simulink model "nmpcSine"  (R2024b)
settings: Solver=FixedStepAuto  StartTime=0.0  StopTime=160  FixedStep=Ts  RelTol=1e-3
model workspace (MAT data in the model file):
  Logfile_Data_Object = ros2bag
  Logfile_Data_Object.FilePath = 'C:\Users\mpilo\Documents\Work\Research Project\Code\Catarob\ROS Implementation\Data\rosbag2_2024_09_20-12_24_11\rosbag2_2024_09_20-12_24_11_0.db3'
  Logfile_Data_Object.AvailableBags = "rosbag2_2024_09_20-12_24_11_0.db3"
  Logfile_Data_Object.StartTime = 1726827851.66
  Logfile_Data_Object.EndTime = 1726828062.45
  Logfile_Data_Object.AvailableTopics = table
  Logfile_Data_Object.AvailableTopics.data{1} = [653; 635; 211; 413; 21112]
  Logfile_Data_Object.AvailableTopics.data{2} = categorical
  Logfile_Data_Object.AvailableTopics.data{2}.categoryNames = {'catarob_interfaces/HullStatus'; 'sensor_msgs/Imu'; 'sensor_msgs/NavSatFix'; 'std_msgs/Float64'}
  Logfile_Data_Object.AvailableTopics.data{2}.codes = [1; 1; 3; 4; 2]
  Logfile_Data_Object.AvailableTopics.data{3}{1} = '
    | int32 status
    | single temp
    | int32 actual_pwm
    | int32 actual_pwm_rc
    | int32 pwm_source
    | single ibat
    | single imot
    | single vbat
    | single actual_imax
    | int32 tor_rc
    | int32 water_ingress
    | int32 pwr_relay'
  Logfile_Data_Object.AvailableTopics.data{3}{2} = '
    | int32 status
    | single temp
    | int32 actual_pwm
    | int32 actual_pwm_rc
    | int32 pwm_source
    | single ibat
    | single imot
    | single vbat
    | single actual_imax
    | int32 tor_rc
    | int32 water_ingress
    | int32 pwr_relay'
  Logfile_Data_Object.AvailableTopics.data{3}{3} = '%
    | % Specified using the WGS 84 reference ellipsoid
    | 
    | % header.stamp specifies the ROS Time for this measurement (the
    | %        corresponding satellite Time may be reported using the
    | %        sensor_msgs/TimeReference message).
    | %
    | % header.frame_id is the frame of reference reported by the satellite
    | %        receiver, usually the location of the antenna.  This is a
    | %        Euclidean frame relative to the vehicle, not a reference
    | %        ellipsoid.
    | std_msgs/Header header
    | 
    | % Satellite fix status information.
    | NavSatStatus status
    | 
    | % Latitude [degrees]. Positive is north of equator; negative is south.
    | double latitude
    | 
    | % Longitude [degrees]. Positive is east of prime meridian; negative is west.
    | double longitude
    | 
    | % Altitude [m]. Positive is above the WGS 84 ellipsoid
    | % (quiet NaN if no altitude is available).
    | double altitude
    | 
    | % Position covariance [m^2] defined relative to a tangential plane
    | % through the reported position. The components are East, North, and
    | % Up (ENU), in row-major order.
    | %
    | % Beware: this coordinate system exhibits singularities at the poles.
    | double[9] position_covariance
    | 
    | % If the covariance of the fix is known, fill it in completely. If the
    | % GPS receiver provides the variance of each measurement, put them
    | % along the diagonal. If only Dilution of Precision is available,
    | % estimate an approximate covariance from that.
    | 
    | uint8 COVARIANCE_TYPEUNKNOWN = 0
    | uint8 COVARIANCE_TYPEAPPROXIMATED = 1
    | uint8 COVARIANCE_TYPE_DIAGONALKNOWN = 2
    | uint8 COVARIANCE_TYPEKNOWN = 3
    | 
    | uint8 position_covariance_type'
  Logfile_Data_Object.AvailableTopics.data{3}{4} = '% It is deprecated as of Foxy
    | % It is recommended to create your own semantically meaningful message.
    | % However if you would like to continue using this please use the equivalent in example_msgs.
    | 
    | double data'
  Logfile_Data_Object.AvailableTopics.data{3}{5} = '%
    | % Accelerations should be in m/s^2 (not in g''s), and rotational velocity should be in rad/sec
    | %
    | % If the covariance of the measurement is known, it should be filled in (if all you know is the
    | % variance of each measurement, e.g. from the datasheet, just put those along the diagonal)
    | % A covariance matrix of all zeros will be interpreted as "covariance unknown", and to use the
    | % data a covariance will have to be assumed or gotten from some other source
    | %
    | % If you have no estimate for one of the data elements (e.g. your IMU doesn''t produce an
    | % orientation estimate), please set element 0 of the associated covariance matrix to -1
    | % If you are interpreting this message, please check for a value of -1 in the first element of each
    | % covariance matrix, and disregard the associated estimate.
    | 
    | std_msgs/Header header
    | 
    | geometry_msgs/Quaternion orientation
    | double[9] orientation_covariance         % Row major about x, y, z axes
    | 
    | geometry_msgs/Vector3 angular_velocity
    | double[9] angular_velocity_covariance    % Row major about x, y, z axes
    | 
    | geometry_msgs/Vector3 linear_acceleration
    | double[9] linear_acceleration_covariance % Row major x, y z'
  Logfile_Data_Object.AvailableTopics.ndims = 2
  Logfile_Data_Object.AvailableTopics.nrows = 5
  Logfile_Data_Object.AvailableTopics.rownames = {'/platform/hull/PORT_status'; '/platform/hull/STBD_status'; '/sensor/emlid_gps_fix'; '/sensors/mag_heading'; '/sensors/ouster/imu'}
  Logfile_Data_Object.AvailableTopics.nvars = 3
  Logfile_Data_Object.AvailableTopics.varnames = {'NumMessages', 'MessageType', 'MessageDefinition'}
  Logfile_Data_Object.AvailableTopics.props.useVariableNamesOriginal = 0
  Logfile_Data_Object.AvailableTopics.props.useDimensionNamesOriginal = 0
  Logfile_Data_Object.AvailableTopics.props.CustomProps = struct()
  Logfile_Data_Object.AvailableTopics.props.VariableCustomProps = struct()
  Logfile_Data_Object.AvailableTopics.props.versionSavedFrom = 4
  Logfile_Data_Object.AvailableTopics.props.minCompatibleVersion = 1
  Logfile_Data_Object.AvailableTopics.props.incompatibilityMsg = ''
  Logfile_Data_Object.AvailableTopics.props.VersionSavedFrom = 4
  Logfile_Data_Object.AvailableTopics.props.Description = ''
  Logfile_Data_Object.AvailableTopics.props.VariableNamesOriginal = {}
  Logfile_Data_Object.AvailableTopics.props.DimensionNames = {'Row', 'Variables'}
  Logfile_Data_Object.AvailableTopics.props.DimensionNamesOriginal = {}
  Logfile_Data_Object.AvailableTopics.props.UserData = []
  Logfile_Data_Object.AvailableTopics.props.VariableDescriptions = {}
  Logfile_Data_Object.AvailableTopics.props.VariableUnits = {}
  Logfile_Data_Object.AvailableTopics.props.VariableContinuity = {}
  Logfile_Data_Object.MessageList = table
  Logfile_Data_Object.MessageList.data{1} = [1726827851.66 1726827851.66 1726827851.67 1726827851.67 1726827851.68 1726827851.69 1726827851.69 1726827851.69 1726827851.7 1726827851.7 1726827851.72 1726827851.72 ... (23024 elements, 23024x1)]
  Logfile_Data_Object.MessageList.data{2} = categorical
  Logfile_Data_Object.MessageList.data{2}.categoryNames = {'/platform/hull/PORT_status'; '/platform/hull/STBD_status'; '/sensor/emlid_gps_fix'; '/sensors/mag_heading'; '/sensors/ouster/imu'}
  Logfile_Data_Object.MessageList.data{2}.codes = [5 5 5 5 5 5 5 5 5 5 5 5 ... (23024 elements, 23024x1)]
  Logfile_Data_Object.MessageList.data{3} = categorical
  Logfile_Data_Object.MessageList.data{3}.categoryNames = {'catarob_interfaces/HullStatus'; 'sensor_msgs/NavSatFix'; 'std_msgs/Float64'; 'sensor_msgs/Imu'}
  Logfile_Data_Object.MessageList.data{3}.codes = [4 4 4 4 4 4 4 4 4 4 4 4 ... (23024 elements, 23024x1)]
  Logfile_Data_Object.MessageList.ndims = 2
  Logfile_Data_Object.MessageList.nrows = 23024
  Logfile_Data_Object.MessageList.nvars = 3
  Logfile_Data_Object.MessageList.varnames = {'Time', 'Topic', 'MessageType'}
  Logfile_Data_Object.MessageList.props.useVariableNamesOriginal = 0
  Logfile_Data_Object.MessageList.props.useDimensionNamesOriginal = 0
  Logfile_Data_Object.MessageList.props.CustomProps = struct()
  Logfile_Data_Object.MessageList.props.VariableCustomProps = struct()
  Logfile_Data_Object.MessageList.props.versionSavedFrom = 4
  Logfile_Data_Object.MessageList.props.minCompatibleVersion = 1
  Logfile_Data_Object.MessageList.props.incompatibilityMsg = ''
  Logfile_Data_Object.MessageList.props.VersionSavedFrom = 4
  Logfile_Data_Object.MessageList.props.Description = ''
  Logfile_Data_Object.MessageList.props.VariableNamesOriginal = {}
  Logfile_Data_Object.MessageList.props.DimensionNames = {'Row', 'Variables'}
  Logfile_Data_Object.MessageList.props.DimensionNamesOriginal = {}
  Logfile_Data_Object.MessageList.props.UserData = []
  Logfile_Data_Object.MessageList.props.VariableDescriptions = {}
  Logfile_Data_Object.MessageList.props.VariableUnits = {}
  Logfile_Data_Object.MessageList.props.VariableContinuity = {}
  Logfile_Data_Object.TopicTypeMap = containers.Map
  Logfile_Data_Object.TopicTypeMap.serialization.keys = {'/platform/hull/PORT_status', '/platform/hull/STBD_status', '/sensor/emlid_gps_fix', '/sensors/mag_heading', '/sensors/ouster/imu'}
  Logfile_Data_Object.TopicTypeMap.serialization.values = {'catarob_interfaces/HullStatus', 'catarob_interfaces/HullStatus', 'sensor_msgs/NavSatFix', 'std_msgs/Float64', 'sensor_msgs/Imu'}
  Logfile_Data_Object.TopicTypeMap.serialization.uniformity = 1
  Logfile_Data_Object.TopicTypeMap.serialization.keyType = 'char'
  Logfile_Data_Object.TopicTypeMap.serialization.valueType = 'char'
  Logfile_Data_Object.TopicDefinitionMap = containers.Map
  Logfile_Data_Object.TopicDefinitionMap.serialization.keys = {'/platform/hull/PORT_status', '/platform/hull/STBD_status', '/sensor/emlid_gps_fix', '/sensors/mag_heading', '/sensors/ouster/imu'}
  Logfile_Data_Object.TopicDefinitionMap.serialization.values{1} = '
    | int32 status
    | single temp
    | int32 actual_pwm
    | int32 actual_pwm_rc
    | int32 pwm_source
    | single ibat
    | single imot
    | single vbat
    | single actual_imax
    | int32 tor_rc
    | int32 water_ingress
    | int32 pwr_relay'
  Logfile_Data_Object.TopicDefinitionMap.serialization.values{2} = '
    | int32 status
    | single temp
    | int32 actual_pwm
    | int32 actual_pwm_rc
    | int32 pwm_source
    | single ibat
    | single imot
    | single vbat
    | single actual_imax
    | int32 tor_rc
    | int32 water_ingress
    | int32 pwr_relay'
  Logfile_Data_Object.TopicDefinitionMap.serialization.values{3} = '%
    | % Specified using the WGS 84 reference ellipsoid
    | 
    | % header.stamp specifies the ROS Time for this measurement (the
    | %        corresponding satellite Time may be reported using the
    | %        sensor_msgs/TimeReference message).
    | %
    | % header.frame_id is the frame of reference reported by the satellite
    | %        receiver, usually the location of the antenna.  This is a
    | %        Euclidean frame relative to the vehicle, not a reference
    | %        ellipsoid.
    | std_msgs/Header header
    | 
    | % Satellite fix status information.
    | NavSatStatus status
    | 
    | % Latitude [degrees]. Positive is north of equator; negative is south.
    | double latitude
    | 
    | % Longitude [degrees]. Positive is east of prime meridian; negative is west.
    | double longitude
    | 
    | % Altitude [m]. Positive is above the WGS 84 ellipsoid
    | % (quiet NaN if no altitude is available).
    | double altitude
    | 
    | % Position covariance [m^2] defined relative to a tangential plane
    | % through the reported position. The components are East, North, and
    | % Up (ENU), in row-major order.
    | %
    | % Beware: this coordinate system exhibits singularities at the poles.
    | double[9] position_covariance
    | 
    | % If the covariance of the fix is known, fill it in completely. If the
    | % GPS receiver provides the variance of each measurement, put them
    | % along the diagonal. If only Dilution of Precision is available,
    | % estimate an approximate covariance from that.
    | 
    | uint8 COVARIANCE_TYPEUNKNOWN = 0
    | uint8 COVARIANCE_TYPEAPPROXIMATED = 1
    | uint8 COVARIANCE_TYPE_DIAGONALKNOWN = 2
    | uint8 COVARIANCE_TYPEKNOWN = 3
    | 
    | uint8 position_covariance_type'
  Logfile_Data_Object.TopicDefinitionMap.serialization.values{4} = '% It is deprecated as of Foxy
    | % It is recommended to create your own semantically meaningful message.
    | % However if you would like to continue using this please use the equivalent in example_msgs.
    | 
    | double data'
  Logfile_Data_Object.TopicDefinitionMap.serialization.values{5} = '%
    | % Accelerations should be in m/s^2 (not in g''s), and rotational velocity should be in rad/sec
    | %
    | % If the covariance of the measurement is known, it should be filled in (if all you know is the
    | % variance of each measurement, e.g. from the datasheet, just put those along the diagonal)
    | % A covariance matrix of all zeros will be interpreted as "covariance unknown", and to use the
    | % data a covariance will have to be assumed or gotten from some other source
    | %
    | % If you have no estimate for one of the data elements (e.g. your IMU doesn''t produce an
    | % orientation estimate), please set element 0 of the associated covariance matrix to -1
    | % If you are interpreting this message, please check for a value of -1 in the first element of each
    | % covariance matrix, and disregard the associated estimate.
    | 
    | std_msgs/Header header
    | 
    | geometry_msgs/Quaternion orientation
    | double[9] orientation_covariance         % Row major about x, y, z axes
    | 
    | geometry_msgs/Vector3 angular_velocity
    | double[9] angular_velocity_covariance    % Row major about x, y, z axes
    | 
    | geometry_msgs/Vector3 linear_acceleration
    | double[9] linear_acceleration_covariance % Row major x, y z'
  Logfile_Data_Object.TopicDefinitionMap.serialization.uniformity = 1
  Logfile_Data_Object.TopicDefinitionMap.serialization.keyType = 'char'
  Logfile_Data_Object.TopicDefinitionMap.serialization.valueType = 'char'
  Logfile_Data_Object.RawMessageBuffer = containers.Map
  Logfile_Data_Object.RawMessageBuffer.serialization.keys = {}
  Logfile_Data_Object.RawMessageBuffer.serialization.values = {}
  Logfile_Data_Object.RawMessageBuffer.serialization.uniformity = 0
  Logfile_Data_Object.RawMessageBuffer.serialization.keyType = 'char'
  Logfile_Data_Object.RawMessageBuffer.serialization.valueType = 'any'
  Logfile_Data_Object.ImgMessageBuffer = containers.Map
  Logfile_Data_Object.ImgMessageBuffer.serialization.keys = {}
  Logfile_Data_Object.ImgMessageBuffer.serialization.values = {}
  Logfile_Data_Object.ImgMessageBuffer.serialization.uniformity = 0
  Logfile_Data_Object.ImgMessageBuffer.serialization.keyType = 'char'
  Logfile_Data_Object.ImgMessageBuffer.serialization.valueType = 'any'
  Logfile_Data_Object.PointCloudBuffer = containers.Map
  Logfile_Data_Object.PointCloudBuffer.serialization.keys = {}
  Logfile_Data_Object.PointCloudBuffer.serialization.values = {}
  Logfile_Data_Object.PointCloudBuffer.serialization.uniformity = 0
  Logfile_Data_Object.PointCloudBuffer.serialization.keyType = 'char'
  Logfile_Data_Object.PointCloudBuffer.serialization.valueType = 'any'
  Logfile_Data_Object.LaserScanBuffer = containers.Map
  Logfile_Data_Object.LaserScanBuffer.serialization.keys = {}
  Logfile_Data_Object.LaserScanBuffer.serialization.values = {}
  Logfile_Data_Object.LaserScanBuffer.serialization.uniformity = 0
  Logfile_Data_Object.LaserScanBuffer.serialization.keyType = 'char'
  Logfile_Data_Object.LaserScanBuffer.serialization.valueType = 'any'
  Logfile_Path = 'C:\Users\mpilo\Documents\Work\Research Project\Code\Catarob\ROS Implementation\Data\rosbag2_2024_09_20-12_24_11\rosbag2_2024_09_20-12_24_11_0.db3'
  Logfile_Playback_Duration = nan
  Logfile_Playback_Offset = nan
values from neighbouring files (symbols this model uses):
  x = X(2:p+1,1)    [costFcn.m]    (also in costFcnJacobian.m = X(2:p+1, 1); stateTransitionFcnJacobianAD.m = x(:))
  y = [x(1);x(2);x(3);x(6)]    [SystemDynamics.m]    (also in costFcn.m = X(2:p+1,2); costFcnJacobian.m = X(2:p+1, 2); gpsMeasurementFcn.m = x([1 2]); imuMeasurementFcn.m = x(6))
undefined symbols (not defined in the file or in its folder): angular, covariance, linear, psi, r, regMdl, Ts, Ts_gps, Ts_mag, v, x_ref2, y_ref2
libraries: ros2lib x12, sharedTrackingLibrary x1, mpclib x1
settings Model: Creator=mpilo  LastModifiedBy=mpilo
settings OptimizationCC: DefaultParameterBehavior=Inlined  EnhancedBackFolding=on  PassReuseOutputArgsAs=Individual arguments  ZeroExternalMemoryAtStartup=off  ZeroInternalMemoryAtStartup=off  MaxStackSize=64  OptimizeBlockOrder=speed  DifferentSizesBufferReuse=on  OptimizationCustomize=off  EfficientTunableParamExpr=on
settings DebuggingCC: ParameterTunabilityLossMsg=error
settings HardwareCC: ProdBitPerLong=64  ProdHWDeviceType=Intel->x86-64 (Linux 64)
settings SFSimCC: MATLABDynamicMemAlloc=off
settings RTWCC: Description=Embedded Coder  SystemTargetFile=ert.tlc  HardwareBoard=Robot Operating System 2 (ROS 2)  TLCOptions="-aInlineSetEventsForThisBaseRateFcn=TLC_FALSE -aSuppressMultiTaskScheduler=TLC_FALSE  -aRateBasedStepFcn=0"  TemplateMakefile=ert_default_tmf  Toolchain=Colcon Tools  TargetLang=C++
settings CodeAppCC: ForceParamTrailComments=on  IgnoreCustomStorageClasses=off  OperatorAnnotations=on  SimulinkDataObjDesc=on  SFDataObjDesc=on  InsertBlockDesc=on
settings ERTTargetCC: CodeInterfacePackaging=C++ class  SupportComplex=off  SupportVariableSizeSignals=on  RootIOFormat=Structure reference

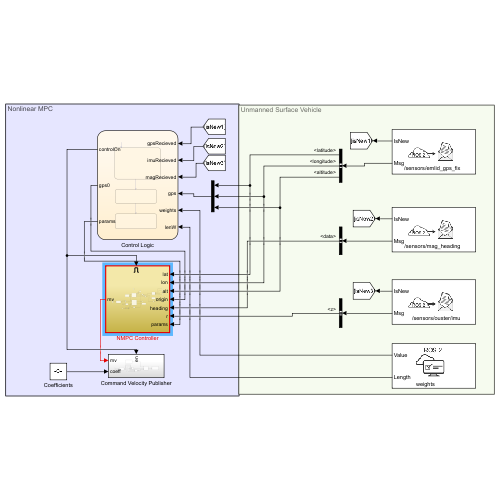
[thumbnail: Simulink's stored preview of the top-level diagram]
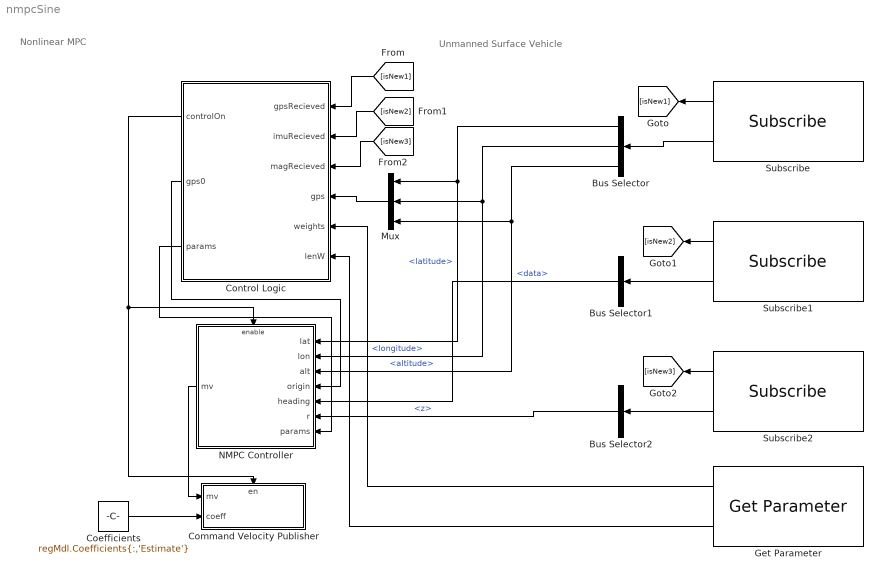
== system nmpcSine ==
  note: Nonlinear MPC
  note: Unmanned Surface Vehicle
  Bus Selector : BusSelector  OutputSignals=latitude,longitude,altitude
  Bus Selector1 : BusSelector  OutputSignals=data
  Bus Selector2 : BusSelector  OutputSignals=angular_velocity.z
  Coefficients : Constant  Value=regMdl.Coefficients{:,'Estimate'}
  Command Velocity Publisher : Subsystem
      settings: PortSchema="{\"entries\":[{\"content\":{\"sides\":[{\"content\":{\"connectorIds\":[\"In1\",\"In2\"]},\"type\":\"ConnectorPlacement.EquallySpacedRectSide\",\"uuid\":\"bfd4065c-1d7a-4c6d-ac5e-0edbc33a7259\"},{\"content\":{\"side\":\"RIGHT\"},\"type\":\"ConnectorPlacement.EquallySpacedRectSide\",\"uuid\":\"c8405d6f-c423-4839-8a94-12941b343a53\"},{\"content\":{\"connectorIds\":[\"In3\"],\"side\":\"TOP\"},\"type\":\"ConnectorPlacement.EquallySpacedRectSide\",\"uuid\":\"7f9aad0c-ddac-4e3c-be3b-f8753d06db0d\"}]},\"type\":\"ConnectorPlacement.EquallySpacedConnector\",\"uuid\":\"a39405ad-bdc0-4278-a227-9b7ebd5e9d6f\"}],\"packageUris\":[\"http://schema.mathworks.com/mf0/Connector/R2020b\"],\"version\":\"1.0\"}"
  Control Logic : Stateflow chart  TreatAsAtomicUnit=on
  Get Parameter : ros2lib/Get Parameter  ParameterName=weights  ParameterType=double[]  ParameterMaxArrayLength=3  ParameterInitialValue=-1  SampleTime=Ts  ModelName=nmpcSine  BlockId=ParamGet_nmpcSine_289
  Mux : Mux  Inputs=3
  NMPC Controller : Subsystem
  Subscribe : ros2lib/Subscribe  topicSource=Specify your own  topic=/sensors/emlid_gps_fix  messageType=sensor_msgs/NavSatFix  sampleTime=Ts_gps  QOSHistory=Keep last  QOSDepth=1  QOSReliability=Best effort  QOSDurability=Volatile  QOSDeadline=Inf  QOSLifespan=Inf  QOSLiveliness=Automatic  QOSLeaseDuration=Inf  QOSAvoidROSNamespaceConventions=off
  Subscribe1 : ros2lib/Subscribe  topicSource=Specify your own  topic=/sensors/mag_heading  messageType=std_msgs/Float64  sampleTime=Ts_mag  QOSHistory=Keep last  QOSDepth=1  QOSReliability=Best effort  QOSDurability=Volatile  QOSDeadline=Inf  QOSLifespan=Inf  QOSLiveliness=Automatic  QOSLeaseDuration=Inf  QOSAvoidROSNamespaceConventions=off
  Subscribe2 : ros2lib/Subscribe  topicSource=Specify your own  topic=/sensors/ouster/imu  messageType=sensor_msgs/Imu  sampleTime=Ts  QOSHistory=Keep last  QOSDepth=1  QOSReliability=Best effort  QOSDurability=Volatile  QOSDeadline=Inf  QOSLifespan=Inf  QOSLiveliness=Automatic  QOSLeaseDuration=Inf  QOSAvoidROSNamespaceConventions=off
  wires:
  Subscribe/1 -> [isNew1]
  Subscribe/2 -> Bus Selector/1
  Bus Selector/3 -> NMPC Controller/3(alt), Mux/3  "<altitude>"
  Bus Selector/2 -> NMPC Controller/2(lon), Mux/2  "<longitude>"
  Bus Selector/1 -> NMPC Controller/1(lat), Mux/1  "<latitude>"
  Subscribe1/2 -> Bus Selector1/1
  Bus Selector1/1 -> NMPC Controller/5(heading)  "<data>"
  Subscribe1/1 -> [isNew2]
  Subscribe2/1 -> [isNew3]
  Subscribe2/2 -> Bus Selector2/1
  Coefficients/1 -> Command Velocity Publisher/2(coeff)
  NMPC Controller/1(mv) -> Command Velocity Publisher/1(mv)
  [isNew1] -> Control Logic/1(gpsRecieved)
  [isNew2] -> Control Logic/2(imuRecieved)
  [isNew3] -> Control Logic/3(magRecieved)
  Control Logic/1(controlOn) -> NMPC Controller/Enable, Command Velocity Publisher/3(en)
  Mux/1 -> Control Logic/4(gps)
  Control Logic/2(gps0) -> NMPC Controller/4(origin)
  Bus Selector2/1 -> NMPC Controller/6(r)  "<z>"
  Get Parameter/2 -> Control Logic/6(lenW)
  Get Parameter/1 -> Control Logic/5(weights)
  Control Logic/3(params) -> NMPC Controller/7(params)

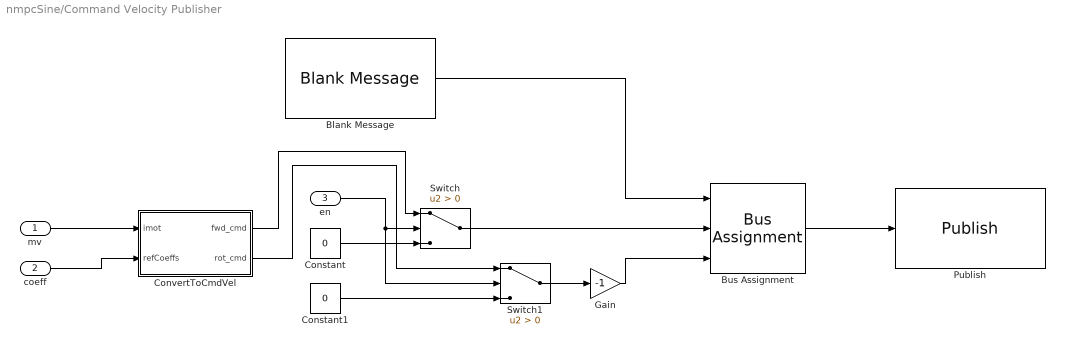
== system nmpcSine/Command Velocity Publisher ==
  mv : Inport
  coeff : Inport  Port=2
  en : Inport  Port=3
  Blank Message : ros2lib/Blank Message  messageClass=Message  entityType=geometry_msgs/Twist  messageType=geometry_msgs/Twist  SampleTime=Ts
  Bus Assignment : BusAssignment  AssignedSignals=linear.x,angular.z
  Constant : Constant  Value=0
  Constant1 : Constant  Value=0
  ConvertToCmdVel : MATLAB Function  TreatAsAtomicUnit=on
  Gain : Gain  Gain=-1
  Publish : ros2lib/Publish  topicSource=Specify your own  topic=/platform/cmd_vel  messageType=geometry_msgs/Twist  QOSHistory=Keep last  QOSDepth=1  QOSReliability=Best effort  QOSDurability=Volatile  QOSDeadline=Inf  QOSLifespan=Inf  QOSLiveliness=Automatic  QOSLeaseDuration=Inf  QOSAvoidROSNamespaceConventions=off
  Switch : Switch  Criteria=u2 > Threshold  SaturateOnIntegerOverflow=off  InputSameDT=off
  Switch1 : Switch  Criteria=u2 > Threshold  SaturateOnIntegerOverflow=off  InputSameDT=off
  wires:
  mv/1 -> ConvertToCmdVel/1(imot)
  Blank Message/1 -> Bus Assignment/1
  Bus Assignment/1 -> Publish/1
  ConvertToCmdVel/1(fwd_cmd) -> Switch/1
  ConvertToCmdVel/2(rot_cmd) -> Switch1/1
  coeff/1 -> ConvertToCmdVel/2(refCoeffs)
  Switch1/1 -> Gain/1
  Switch/1 -> Bus Assignment/2
  en/1 -> Switch1/2, Switch/2
  Constant/1 -> Switch/3
  Constant1/1 -> Switch1/3
  Gain/1 -> Bus Assignment/3

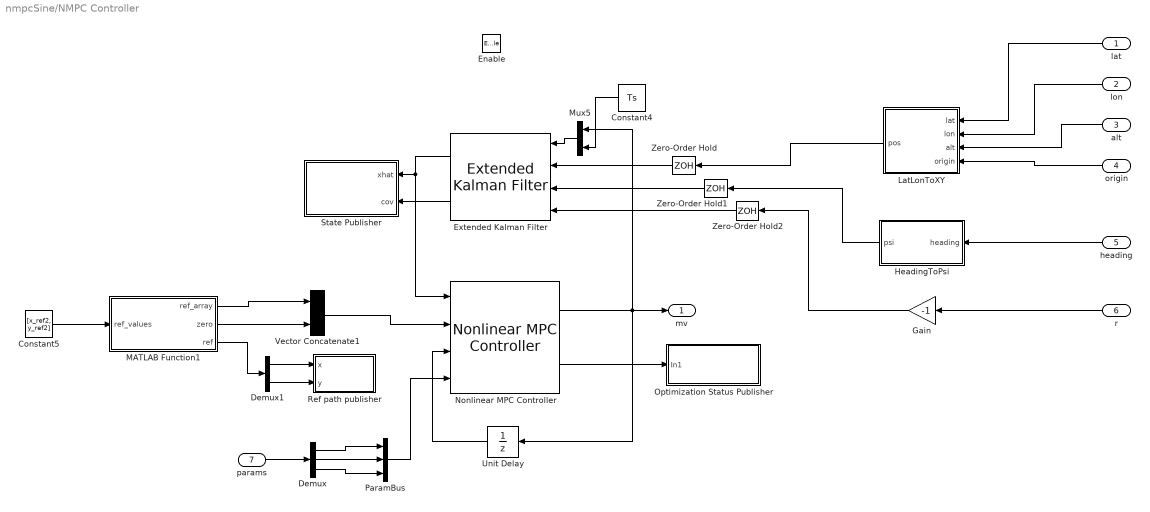
== system nmpcSine/NMPC Controller ==
  lat : Inport
  lon : Inport  Port=2
  alt : Inport  Port=3
  origin : Inport  Port=4
  heading : Inport  Port=5
  r : Inport  Port=6
  params : Inport  Port=7
  Enable : EnablePort
  Constant4 : Constant  Value=Ts  SampleTime=Ts
  Constant5 : Constant  Value=[x_ref2, y_ref2]  SampleTime=Ts
  Demux : Demux  Outputs=3
  Demux1 : Demux  Outputs=2
  Extended Kalman Filter : sharedTrackingLibrary/Extended Kalman Filter  StateTransitionFcn=stateTransitionFcnDT  HasStateTransitionJacobianFcn=off  StateTransitionJacobianFcn=stateTransitionFcnJacobian  HasAdditiveProcessNoise=Additive  ProcessNoise=Q  HasTimeVaryingProcessNoise=off  HasStateTransitionFcnExtraArgument=1  InitialState=x0  InitialStateCovariance=P_0  MeasurementFcn1=gpsMeasurementFcn  HasMeasurementJacobianFcn1=off  HasMeasurementEnablePort1=off  HasAdditiveMeasurementNoise1=Additive  MeasurementNoise1=R_gps  HasTimeVaryingMeasurementNoise1=off  HasMeasurementFcnExtraArgument1=0  HasMeasurementWrapping1=off  MeasurementFcn2=magMeasurementFcn  HasMeasurementJacobianFcn2=off  HasMeasurementEnablePort2=off  HasAdditiveMeasurementNoise2=Additive  MeasurementNoise2=R_mag  HasTimeVaryingMeasurementNoise2=off  HasMeasurementFcnExtraArgument2=0  HasMeasurementWrapping2=on  MeasurementFcn3=imuMeasurementFcn  HasMeasurementJacobianFcn3=off  HasMeasurementEnablePort3=off  HasAdditiveMeasurementNoise3=Additive  MeasurementNoise3=R_imu  HasTimeVaryingMeasurementNoise3=off  HasMeasurementFcnExtraArgument3=0  HasMeasurementWrapping3=off  MeasurementFcn4=myMeasurementFcn  HasMeasurementJacobianFcn4=off  HasMeasurementEnablePort4=off  HasAdditiveMeasurementNoise4=Additive  MeasurementNoise4=1  HasTimeVaryingMeasurementNoise4=off  HasMeasurementFcnExtraArgument4=0  HasMeasurementWrapping4=off  MeasurementFcn5=myMeasurementFcn  HasMeasurementJacobianFcn5=off  HasMeasurementEnablePort5=off  HasAdditiveMeasurementNoise5=Additive  MeasurementNoise5=1  HasTimeVaryingMeasurementNoise5=off  HasMeasurementFcnExtraArgument5=0  HasMeasurementWrapping5=off  EnableMultirate=on  StateTransitionFcnSampleTime=Ts  MeasurementFcn1SampleTime=Ts_gps  MeasurementFcn2SampleTime=Ts_mag  MeasurementFcn3SampleTime=Ts  MeasurementFcn4SampleTime=1  MeasurementFcn5SampleTime=1  UseCurrentEstimator=on  OutputStateCovariance=on  DataType=double  SampleTime=1  NumberOfMeasurements=3
      settings: LibrarySourceBlock=slident/Estimators/Extended Kalman Filter
  Gain : Gain  Gain=-1
  HeadingToPsi : MATLAB Function  TreatAsAtomicUnit=on
  LatLonToXY : MATLAB Function  TreatAsAtomicUnit=on
  MATLAB Function1 : MATLAB Function  TreatAsAtomicUnit=on
  Mux5 : Mux  Inputs=2
  Nonlinear MPC Controller : mpclib/Nonlinear MPC Controller  nlmpcobj=nlobj  UseObjectTs=on  UseMEX=off  mexname=nmpcController  md_enabled=off  mvtarget_enabled=off  param_enabled=on  cost_enabled=off  mvseq_enabled=off  stateseq_enabled=off  ovseq_enabled=off  slack_enabled=off  status_enabled=on  ov_min=off  ov_max=off  mv_min=off  mv_max=off  mvrate_min=off  mvrate_max=off  state_min=off  state_max=off  ov_weight=off  mv_weight=off  mvrate_weight=off  ecr_weight=off  nlp_initialize=off
  Optimization Status Publisher : Subsystem
  ParamBus : BusCreator  Inputs=3  OutDataTypeStr=Bus: ParamBus  NonVirtualBus=on
      settings: InheritFromInputs=off
  Ref path publisher : Subsystem
  State Publisher : Subsystem
  Unit Delay : UnitDelay  InitialCondition=[0;0]  SampleTime=Ts  HasFrameUpgradeWarning=on
  Vector Concatenate1 : Concatenate  Mode=Multidimensional array  ConcatenateDimension=2
  Zero-Order Hold : ZeroOrderHold  SampleTime=Ts_gps
  Zero-Order Hold1 : ZeroOrderHold  SampleTime=Ts_mag
  Zero-Order Hold2 : ZeroOrderHold  SampleTime=Ts
  mv : Outport
  wires:
  Zero-Order Hold2/1 -> Extended Kalman Filter/4
  Nonlinear MPC Controller/1 -> Unit Delay/1, mv/1, Mux5/1
  Constant4/1 -> Mux5/2
  Mux5/1 -> Extended Kalman Filter/1
  ParamBus/1 -> Nonlinear MPC Controller/4
  Demux/2 -> ParamBus/2
  Zero-Order Hold/1 -> Extended Kalman Filter/2
  Demux/1 -> ParamBus/1
  Extended Kalman Filter/1 -> Nonlinear MPC Controller/1, State Publisher/1(xhat)
  Unit Delay/1 -> Nonlinear MPC Controller/3
  Zero-Order Hold1/1 -> Extended Kalman Filter/3
  Extended Kalman Filter/2 -> State Publisher/2(cov)
  Nonlinear MPC Controller/2 -> Optimization Status Publisher/1(In1)
  lat/1 -> LatLonToXY/1(lat)
  lon/1 -> LatLonToXY/2(lon)
  alt/1 -> LatLonToXY/3(alt)
  origin/1 -> LatLonToXY/4(origin)
  LatLonToXY/1(pos) -> Zero-Order Hold/1
  HeadingToPsi/1(psi) -> Zero-Order Hold1/1
  heading/1 -> HeadingToPsi/1(heading)
  r/1 -> Gain/1
  Gain/1 -> Zero-Order Hold2/1
  Demux/3 -> ParamBus/3
  params/1 -> Demux/1
  Vector Concatenate1/1 -> Nonlinear MPC Controller/2
  Demux1/2 -> Ref path publisher/2(y)
  Constant5/1 -> MATLAB Function1/1(ref_values)
  MATLAB Function1/3(ref) -> Demux1/1
  MATLAB Function1/1(ref_array) -> Vector Concatenate1/1
  Demux1/1 -> Ref path publisher/1(x)
  MATLAB Function1/2(zero) -> Vector Concatenate1/2

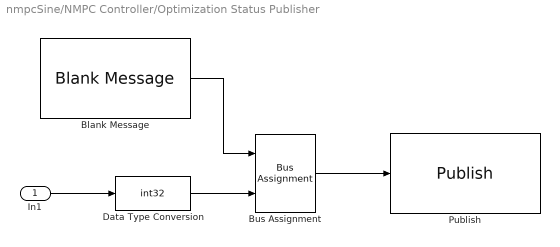
== system nmpcSine/NMPC Controller/Optimization Status Publisher ==
  In1 : Inport
  Blank Message : ros2lib/Blank Message  messageClass=Message  entityType=std_msgs/Int32  messageType=std_msgs/Int32  SampleTime=Ts
  Bus Assignment : BusAssignment  AssignedSignals=data
  Data Type Conversion : DataTypeConversion  OutDataTypeStr=int32  RndMeth=Floor
  Publish : ros2lib/Publish  topicSource=Specify your own  topic=/controller/opt_status  messageType=std_msgs/Int32  QOSHistory=Keep last  QOSDepth=1  QOSReliability=Best effort  QOSDurability=Volatile  QOSDeadline=Inf  QOSLifespan=Inf  QOSLiveliness=Automatic  QOSLeaseDuration=Inf  QOSAvoidROSNamespaceConventions=off
  wires:
  In1/1 -> Data Type Conversion/1
  Blank Message/1 -> Bus Assignment/1
  Data Type Conversion/1 -> Bus Assignment/2
  Bus Assignment/1 -> Publish/1

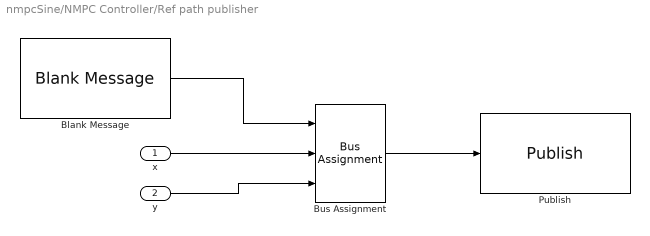
== system nmpcSine/NMPC Controller/Ref path publisher ==
  x : Inport
  y : Inport  Port=2
  Blank Message : ros2lib/Blank Message  messageClass=Message  entityType=geometry_msgs/Point  messageType=geometry_msgs/Point  SampleTime=Ts
  Bus Assignment : BusAssignment  AssignedSignals=x,y
  Publish : ros2lib/Publish  topicSource=Specify your own  topic=/controller/ref_path  messageType=geometry_msgs/Point  QOSHistory=Keep last  QOSDepth=1  QOSReliability=Best effort  QOSDurability=Volatile  QOSDeadline=Inf  QOSLifespan=Inf  QOSLiveliness=Automatic  QOSLeaseDuration=Inf  QOSAvoidROSNamespaceConventions=off
  wires:
  Blank Message/1 -> Bus Assignment/1
  x/1 -> Bus Assignment/2
  y/1 -> Bus Assignment/3
  Bus Assignment/1 -> Publish/1

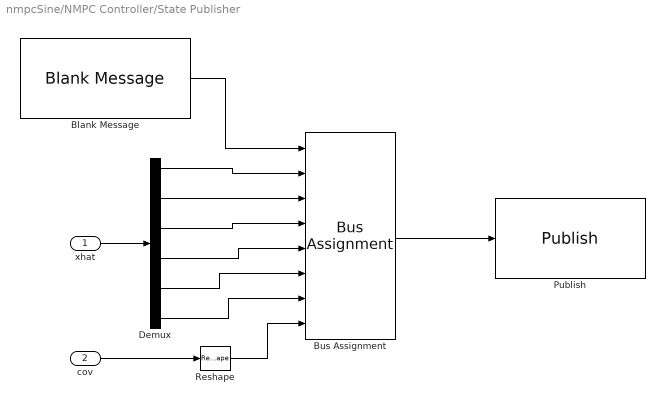
== system nmpcSine/NMPC Controller/State Publisher ==
  xhat : Inport
  cov : Inport  Port=2
  Blank Message : ros2lib/Blank Message  messageClass=Message  entityType=catarob_interfaces/StateEstimate  messageType=catarob_interfaces/StateEstimate  SampleTime=Ts
  Bus Assignment : BusAssignment  AssignedSignals=x,y,psi,u,v,r,covariance
  Demux : Demux  Outputs=6
  Publish : ros2lib/Publish  topicSource=Specify your own  topic=/controller/states  messageType=catarob_interfaces/StateEstimate  QOSHistory=Keep last  QOSDepth=1  QOSReliability=Best effort  QOSDurability=Volatile  QOSDeadline=Inf  QOSLifespan=Inf  QOSLiveliness=Automatic  QOSLeaseDuration=Inf  QOSAvoidROSNamespaceConventions=off
  Reshape : Reshape
  wires:
  xhat/1 -> Demux/1
  Blank Message/1 -> Bus Assignment/1
  Demux/1 -> Bus Assignment/2
  Demux/2 -> Bus Assignment/3
  Demux/3 -> Bus Assignment/4
  Demux/4 -> Bus Assignment/5
  Demux/5 -> Bus Assignment/6
  Demux/6 -> Bus Assignment/7
  cov/1 -> Reshape/1
  Reshape/1 -> Bus Assignment/8
  Bus Assignment/1 -> Publish/1

== matlab function nmpcSine/NMPC Controller/HeadingToPsi ==
  data: heading input; psi output
function psi = fcn(heading)

declination = 26.566667;
psi = deg2rad(wrapTo360(heading - declination));

== matlab function nmpcSine/NMPC Controller/LatLonToXY ==
  data: lat input; pos output; lon input; alt input; origin input
function pos = fcn(lat, lon, alt, origin)

[y,x] = latlon2local(lat, lon, alt, origin);
pos = [x;y];

== matlab function nmpcSine/Command Velocity Publisher/ConvertToCmdVel ==
  data: imot input; fwd_cmd output; rot_cmd output; refCoeffs input
function [fwd_cmd, rot_cmd]   = fcn(imot, refCoeffs)

pwm = refCoeffs(1) + refCoeffs(2)*imot;
pwm = min(255, max(0, pwm));
port_pwm = pwm(1); stbd_pwm = pwm(2);

% Convert PWM values back to velocities
stbd_vel = 2 - (4 * (255 - stbd_pwm) / 255);
port_vel = 2 - (4 * (255 - port_pwm) / 255);

% Calculate forward command (fwd_cmd) and rotational velocity (rot_vel)
fwd_cmd = (stbd_vel + port_vel) / 2;
rot_vel = (port_vel - stbd_vel) / (2 * 0.42);

% Calculate rotational command (rot_cmd)
rot_cmd = rot_vel * 0.42;

== stateflow chart nmpcSine/Control Logic ==
  state Wait
    entry:
    controlOn = 0; en1=0; en2=0; en3=0; gps0 = [0;0;0];
    during:
    if gpsRecieved == 1
    en1 = 1;
    end
    if magRecieved == 1
    en2 = 1;
    end
    if imuRecieved == 1
    en3 = 1;
    end
  state Control
    entry:
    gps0 = gps;
    params = weights.';
    controlOn = 1;
  state Stop
    entry:
    controlOn = 0;
  (default) -> Wait
  Wait -> Control : [en1&en2&en3& lenW == 3]
  Control -> Stop : after(150, sec)
  data: gpsRecieved input; imuRecieved input; magRecieved input; controlOn output; en1 local; en2 local; en3 local; gps input; gps0 output; weights input; lenW input; params output

== matlab function nmpcSine/NMPC Controller/MATLAB Function1 ==
  data: ref_array output; zero output; ref output; ref_values input
function [ref_array, zero, ref] = pathPlanner(ref_values)
%% Sets Reference values for NMPC controller
% ref_values: Matrix of reference values with two columns [x, y]

% Current timestep
persistent k 
if isempty(k)
    k = 1;
end

% p: Number of future values to output (including the current value)
% i.e. Predicition horizon
p = 20;

% Get the number of rows (samples) in the reference array
N = size(ref_values, 1);

% Initialise the output array (p rows for p future values, 
% 2 columns for x and y)
ref = [0;0];
ref_array = zeros(p, 2);
zero = ref_array;  % Output a zero matrix of the same size for psi and r

% Loop through and fill the array with current and next p-1 values
for i = 0:(p-1)
    % Calculate the index for current value and next p-1 values
    % Using modulo operation to loop back around
    idx = mod(k + i - 1, N) + 1;
    
    % Output current reference value for publisher
    if i==0
        ref = transpose(ref_values(idx, :));
    end
    
    % Assign [x, y] values at index idx
    ref_array(i+1, :) = ref_values(idx, :); 
end

% Increment the timestep
k = k + 1;
end
